simulink model "brainstorm_service"  (R2024a)
settings: Solver=FixedStepDiscrete  StartTime=0.0  StopTime=10.0  RelTol=1e-3
model workspace (MAT data in the model file):
  Anatomy = Simulink.ServiceBus
  Anatomy.Elements_internal(1) = Simulink.FunctionElement
  Anatomy.Elements_internal(1).Prototype = 'GetSubjectMri(bst_fullfile,sessFolders,anat)'
  Anatomy.Elements_internal(1).Name = 'GetSubjectMri'
  Anatomy.Elements_internal(1).Asynchronous = 0
  Anatomy.Elements_internal(1).Arguments(1) = Simulink.BusElement
  Anatomy.Elements_internal(1).Arguments(1).DimensionsMode = 'Fixed'
  Anatomy.Elements_internal(1).Arguments(1).SamplingMode = 'Sample based'
  Anatomy.Elements_internal(1).Arguments(1).SampleTime = -1
  Anatomy.Elements_internal(1).Arguments(1).Name = 'bst_fullfile'
  Anatomy.Elements_internal(1).Arguments(1).DataType_internal = 'double'
  Anatomy.Elements_internal(1).Arguments(1).Complexity = 'real'
  Anatomy.Elements_internal(1).Arguments(1).Dimensions = 1
  Anatomy.Elements_internal(1).Arguments(2) = Simulink.BusElement
  Anatomy.Elements_internal(1).Arguments(2).DimensionsMode = 'Fixed'
  Anatomy.Elements_internal(1).Arguments(2).SamplingMode = 'Sample based'
  Anatomy.Elements_internal(1).Arguments(2).SampleTime = -1
  Anatomy.Elements_internal(1).Arguments(2).Name = 'sessFolders'
  Anatomy.Elements_internal(1).Arguments(2).DataType_internal = 'double'
  Anatomy.Elements_internal(1).Arguments(2).Complexity = 'real'
  Anatomy.Elements_internal(1).Arguments(2).Dimensions = 1
  Anatomy.Elements_internal(1).Arguments(3) = Simulink.BusElement
  Anatomy.Elements_internal(1).Arguments(3).DimensionsMode = 'Fixed'
  Anatomy.Elements_internal(1).Arguments(3).SamplingMode = 'Sample based'
  Anatomy.Elements_internal(1).Arguments(3).SampleTime = -1
  Anatomy.Elements_internal(1).Arguments(3).Name = 'anat'
  Anatomy.Elements_internal(1).Arguments(3).DataType_internal = 'double'
  Anatomy.Elements_internal(1).Arguments(3).Complexity = 'real'
  Anatomy.Elements_internal(1).Arguments(3).Dimensions = 1
  Anatomy.Elements_internal(2) = Simulink.FunctionElement
  Anatomy.Elements_internal(2).Prototype = 'SubjectMriFiles()'
  Anatomy.Elements_internal(2).Name = 'SubjectMriFiles'
  Anatomy.Elements_internal(2).Asynchronous = 0
  coregister = Simulink.ServiceBus
  coregister.Elements_internal = Simulink.FunctionElement
  coregister.Elements_internal.Prototype = 'GetFiducials(json,voxel)'
  coregister.Elements_internal.Name = 'GetFiducials'
  coregister.Elements_internal.Asynchronous = 0
  coregister.Elements_internal.Arguments(1) = Simulink.BusElement
  coregister.Elements_internal.Arguments(1).DimensionsMode = 'Fixed'
  coregister.Elements_internal.Arguments(1).SamplingMode = 'Sample based'
  coregister.Elements_internal.Arguments(1).SampleTime = -1
  coregister.Elements_internal.Arguments(1).Name = 'json'
  coregister.Elements_internal.Arguments(1).DataType_internal = 'double'
  coregister.Elements_internal.Arguments(1).Complexity = 'real'
  coregister.Elements_internal.Arguments(1).Dimensions = 1
  coregister.Elements_internal.Arguments(2) = Simulink.BusElement
  coregister.Elements_internal.Arguments(2).DimensionsMode = 'Fixed'
  coregister.Elements_internal.Arguments(2).SamplingMode = 'Sample based'
  coregister.Elements_internal.Arguments(2).SampleTime = -1
  coregister.Elements_internal.Arguments(2).Name = 'voxel'
  coregister.Elements_internal.Arguments(2).DataType_internal = 'double'
  coregister.Elements_internal.Arguments(2).Complexity = 'real'
  coregister.Elements_internal.Arguments(2).Dimensions = 1
  filePaths = Simulink.ServiceBus
  filePaths.Elements_internal(1) = Simulink.FunctionElement
  filePaths.Elements_internal(1).Prototype = 'bst_fullfile(fPath,fBase,json)'
  filePaths.Elements_internal(1).Name = 'bst_fullfile'
  filePaths.Elements_internal(1).Asynchronous = 0
  filePaths.Elements_internal(1).Arguments(1) = Simulink.BusElement
  filePaths.Elements_internal(1).Arguments(1).DimensionsMode = 'Fixed'
  filePaths.Elements_internal(1).Arguments(1).SamplingMode = 'Sample based'
  filePaths.Elements_internal(1).Arguments(1).SampleTime = -1
  filePaths.Elements_internal(1).Arguments(1).Name = 'fPath'
  filePaths.Elements_internal(1).Arguments(1).DataType_internal = 'double'
  filePaths.Elements_internal(1).Arguments(1).Complexity = 'real'
  filePaths.Elements_internal(1).Arguments(1).Dimensions = 1
  filePaths.Elements_internal(1).Arguments(2) = Simulink.BusElement
  filePaths.Elements_internal(1).Arguments(2).DimensionsMode = 'Fixed'
  filePaths.Elements_internal(1).Arguments(2).SamplingMode = 'Sample based'
  filePaths.Elements_internal(1).Arguments(2).SampleTime = -1
  filePaths.Elements_internal(1).Arguments(2).Name = 'fBase'
  filePaths.Elements_internal(1).Arguments(2).DataType_internal = 'double'
  filePaths.Elements_internal(1).Arguments(2).Complexity = 'real'
  filePaths.Elements_internal(1).Arguments(2).Dimensions = 1
  filePaths.Elements_internal(1).Arguments(3) = Simulink.BusElement
  filePaths.Elements_internal(1).Arguments(3).DimensionsMode = 'Fixed'
  filePaths.Elements_internal(1).Arguments(3).SamplingMode = 'Sample based'
  filePaths.Elements_internal(1).Arguments(3).SampleTime = -1
  filePaths.Elements_internal(1).Arguments(3).Name = 'json'
  filePaths.Elements_internal(1).Arguments(3).DataType_internal = 'double'
  filePaths.Elements_internal(1).Arguments(3).Complexity = 'real'
  filePaths.Elements_internal(1).Arguments(3).Dimensions = 1
  filePaths.Elements_internal(2) = Simulink.FunctionElement
  filePaths.Elements_internal(2).Prototype = 'bst_fileparts()'
  filePaths.Elements_internal(2).Name = 'bst_fileparts'
  filePaths.Elements_internal(2).Asynchronous = 0
  importVolume = Simulink.ServiceBus
  importVolume.Elements_internal(1) = Simulink.FunctionElement
  importVolume.Elements_internal(1).Prototype = 'process_import_bids(ImportBidsDataset)'
  importVolume.Elements_internal(1).Name = 'process_import_bids'
  importVolume.Elements_internal(1).Asynchronous = 0
  importVolume.Elements_internal(1).Arguments = Simulink.BusElement
  importVolume.Elements_internal(1).Arguments.DimensionsMode = 'Fixed'
  importVolume.Elements_internal(1).Arguments.SamplingMode = 'Sample based'
  importVolume.Elements_internal(1).Arguments.SampleTime = -1
  importVolume.Elements_internal(1).Arguments.Name = 'ImportBidsDataset'
  importVolume.Elements_internal(1).Arguments.DataType_internal = 'double'
  importVolume.Elements_internal(1).Arguments.Complexity = 'real'
  importVolume.Elements_internal(1).Arguments.Dimensions = 1
  importVolume.Elements_internal(2) = Simulink.FunctionElement
  importVolume.Elements_internal(2).Prototype = 'ImportBidsDataset(BidsDir,OPTIONS)'
  importVolume.Elements_internal(2).Name = 'ImportBidsDataset'
  importVolume.Elements_internal(2).Asynchronous = 0
  importVolume.Elements_internal(2).Arguments(1) = Simulink.BusElement
  importVolume.Elements_internal(2).Arguments(1).DimensionsMode = 'Fixed'
  importVolume.Elements_internal(2).Arguments(1).SamplingMode = 'Sample based'
  importVolume.Elements_internal(2).Arguments(1).SampleTime = -1
  importVolume.Elements_internal(2).Arguments(1).Name = 'BidsDir'
  importVolume.Elements_internal(2).Arguments(1).DataType_internal = 'double'
  importVolume.Elements_internal(2).Arguments(1).Complexity = 'real'
  importVolume.Elements_internal(2).Arguments(1).Dimensions = 1
  importVolume.Elements_internal(2).Arguments(2) = Simulink.BusElement
  importVolume.Elements_internal(2).Arguments(2).DimensionsMode = 'Fixed'
  importVolume.Elements_internal(2).Arguments(2).SamplingMode = 'Sample based'
  importVolume.Elements_internal(2).Arguments(2).SampleTime = -1
  importVolume.Elements_internal(2).Arguments(2).Name = 'OPTIONS'
  importVolume.Elements_internal(2).Arguments(2).DataType_internal = 'double'
  importVolume.Elements_internal(2).Arguments(2).Complexity = 'real'
  importVolume.Elements_internal(2).Arguments(2).Dimensions = 1
  importVolume.Elements_internal(3) = Simulink.FunctionElement
  importVolume.Elements_internal(3).Prototype = 'GetSubjectMri(bst_fullfile,sessFolders,isess,anat)'
  importVolume.Elements_internal(3).Name = 'GetSubjectMri'
  importVolume.Elements_internal(3).Asynchronous = 0
  importVolume.Elements_internal(3).Arguments(1) = Simulink.BusElement
  importVolume.Elements_internal(3).Arguments(1).DimensionsMode = 'Fixed'
  importVolume.Elements_internal(3).Arguments(1).SamplingMode = 'Sample based'
  importVolume.Elements_internal(3).Arguments(1).SampleTime = -1
  importVolume.Elements_internal(3).Arguments(1).Name = 'bst_fullfile'
  importVolume.Elements_internal(3).Arguments(1).DataType_internal = 'double'
  importVolume.Elements_internal(3).Arguments(1).Complexity = 'real'
  importVolume.Elements_internal(3).Arguments(1).Dimensions = 1
  importVolume.Elements_internal(3).Arguments(2) = Simulink.BusElement
  importVolume.Elements_internal(3).Arguments(2).DimensionsMode = 'Fixed'
  importVolume.Elements_internal(3).Arguments(2).SamplingMode = 'Sample based'
  importVolume.Elements_internal(3).Arguments(2).SampleTime = -1
  importVolume.Elements_internal(3).Arguments(2).Name = 'sessFolders'
  importVolume.Elements_internal(3).Arguments(2).DataType_internal = 'double'
  importVolume.Elements_internal(3).Arguments(2).Complexity = 'real'
  importVolume.Elements_internal(3).Arguments(2).Dimensions = 1
  importVolume.Elements_internal(3).Arguments(3) = Simulink.BusElement
  importVolume.Elements_internal(3).Arguments(3).DimensionsMode = 'Fixed'
  importVolume.Elements_internal(3).Arguments(3).SamplingMode = 'Sample based'
  importVolume.Elements_internal(3).Arguments(3).SampleTime = -1
  importVolume.Elements_internal(3).Arguments(3).Name = 'isess'
  importVolume.Elements_internal(3).Arguments(3).DataType_internal = 'double'
  importVolume.Elements_internal(3).Arguments(3).Complexity = 'real'
  importVolume.Elements_internal(3).Arguments(3).Dimensions = 1
  importVolume.Elements_internal(3).Arguments(4) = Simulink.BusElement
  importVolume.Elements_internal(3).Arguments(4).DimensionsMode = 'Fixed'
  importVolume.Elements_internal(3).Arguments(4).SamplingMode = 'Sample based'
  importVolume.Elements_internal(3).Arguments(4).SampleTime = -1
  importVolume.Elements_internal(3).Arguments(4).Name = 'anat'
  importVolume.Elements_internal(3).Arguments(4).DataType_internal = 'double'
  importVolume.Elements_internal(3).Arguments(4).Complexity = 'real'
  importVolume.Elements_internal(3).Arguments(4).Dimensions = 1
  importVolume.Elements_internal(4) = Simulink.FunctionElement
  importVolume.Elements_internal(4).Prototype = 'GetSubjectSeg(BidsDir,subjName,sessDir,isess,name)'
  importVolume.Elements_internal(4).Name = 'GetSubjectSeg'
  importVolume.Elements_internal(4).Asynchronous = 0
  importVolume.Elements_internal(4).Arguments(1) = Simulink.BusElement
  importVolume.Elements_internal(4).Arguments(1).DimensionsMode = 'Fixed'
  importVolume.Elements_internal(4).Arguments(1).SamplingMode = 'Sample based'
  importVolume.Elements_internal(4).Arguments(1).SampleTime = -1
  importVolume.Elements_internal(4).Arguments(1).Name = 'BidsDir'
  importVolume.Elements_internal(4).Arguments(1).DataType_internal = 'double'
  importVolume.Elements_internal(4).Arguments(1).Complexity = 'real'
  importVolume.Elements_internal(4).Arguments(1).Dimensions = 1
  importVolume.Elements_internal(4).Arguments(2) = Simulink.BusElement
  importVolume.Elements_internal(4).Arguments(2).DimensionsMode = 'Fixed'
  importVolume.Elements_internal(4).Arguments(2).SamplingMode = 'Sample based'
  importVolume.Elements_internal(4).Arguments(2).SampleTime = -1
  importVolume.Elements_internal(4).Arguments(2).Name = 'subjName'
  importVolume.Elements_internal(4).Arguments(2).DataType_internal = 'double'
  importVolume.Elements_internal(4).Arguments(2).Complexity = 'real'
  importVolume.Elements_internal(4).Arguments(2).Dimensions = 1
  importVolume.Elements_internal(4).Arguments(3) = Simulink.BusElement
  importVolume.Elements_internal(4).Arguments(3).DimensionsMode = 'Fixed'
  importVolume.Elements_internal(4).Arguments(3).SamplingMode = 'Sample based'
  importVolume.Elements_internal(4).Arguments(3).SampleTime = -1
  importVolume.Elements_internal(4).Arguments(3).Name = 'sessDir'
  importVolume.Elements_internal(4).Arguments(3).DataType_internal = 'double'
  importVolume.Elements_internal(4).Arguments(3).Complexity = 'real'
  importVolume.Elements_internal(4).Arguments(3).Dimensions = 1
  importVolume.Elements_internal(4).Arguments(4) = Simulink.BusElement
  importVolume.Elements_internal(4).Arguments(4).DimensionsMode = 'Fixed'
  importVolume.Elements_internal(4).Arguments(4).SamplingMode = 'Sample based'
  importVolume.Elements_internal(4).Arguments(4).SampleTime = -1
  importVolume.Elements_internal(4).Arguments(4).Name = 'isess'
  importVolume.Elements_internal(4).Arguments(4).DataType_internal = 'double'
  importVolume.Elements_internal(4).Arguments(4).Complexity = 'real'
  importVolume.Elements_internal(4).Arguments(4).Dimensions = 1
  importVolume.Elements_internal(4).Arguments(5) = Simulink.BusElement
  importVolume.Elements_internal(4).Arguments(5).DimensionsMode = 'Fixed'
  importVolume.Elements_internal(4).Arguments(5).SamplingMode = 'Sample based'
  importVolume.Elements_internal(4).Arguments(5).SampleTime = -1
  importVolume.Elements_internal(4).Arguments(5).Name = 'name'
  importVolume.Elements_internal(4).Arguments(5).DataType_internal = 'double'
  importVolume.Elements_internal(4).Arguments(5).Complexity = 'real'
  importVolume.Elements_internal(4).Arguments(5).Dimensions = 1
settings Model: Creator=diell  LastModifiedBy=diell

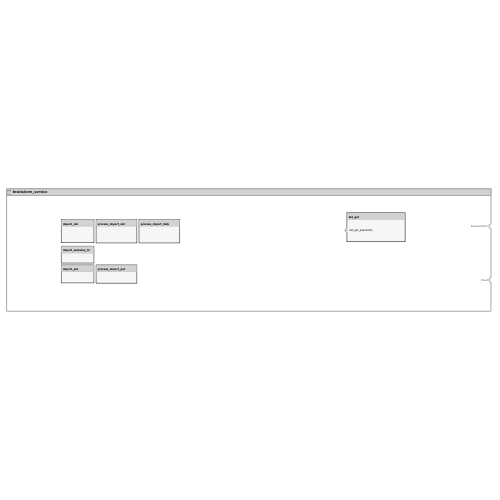
[thumbnail: Simulink's stored preview of the top-level diagram]
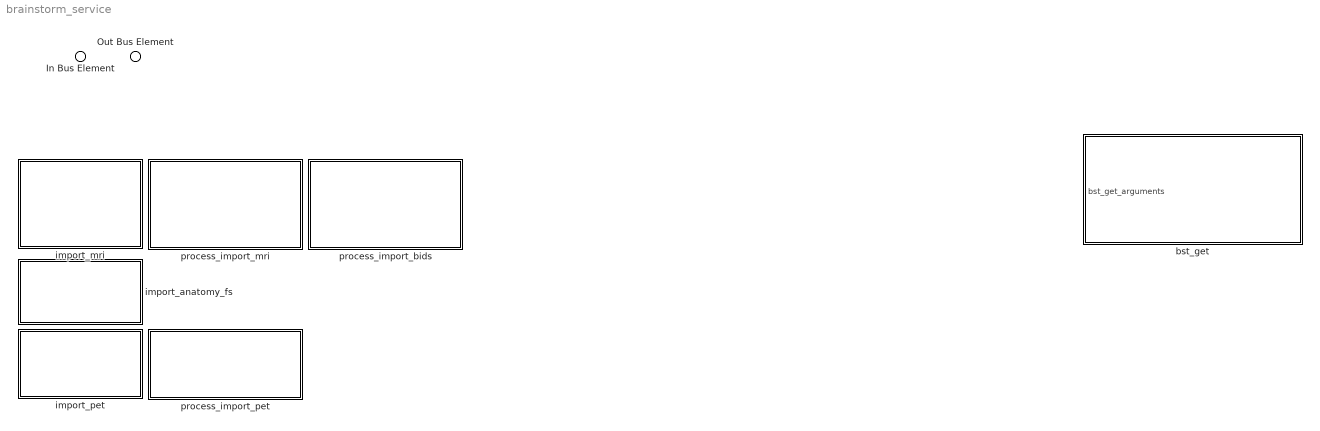
== system brainstorm_service ==
  In Bus Element : Inport  AllowServiceAccess=on  PortName=Client
  bst_get : Subsystem
      settings: PortSchema="{\"entries\":[{\"content\":{\"headerSize\":26,\"margin\":15,\"minimumSpacing\":25,\"sides\":[{\"content\":{\"connectorIds\":[\"In1\"]},\"type\":\"ConnectorPlacement.EquallySpacedRectSide\",\"uuid\":\"7074e736-93ca-48e6-9107-0c0acde2c1e1\"},{\"content\":{\"side\":\"RIGHT\"},\"type\":\"ConnectorPlacement.EquallySpacedRectSide\",\"uuid\":\"49ca3538-4b0a-47e3-9b9f-d0d67086357c\"},{\"content\":{\"side\":\"TOP\"},\"type\":\"ConnectorPlacement.EquallySpacedRectSide\",\"uuid\":\"104f6ef2-0cbf-4c6c-8b7e-db8a41d08c3b\"}]},\"type\":\"ConnectorPlacement.EquallySpacedConnector\",\"uuid\":\"4cd04038-0b55-4958-ad0a-aa155b20eca4\"}],\"packageUris\":[\"http://schema.mathworks.com/mf0/Connector/R2020b\"],\"version\":\"1.0\"}"
  import_anatomy_fs : Subsystem
      settings: PortSchema="{\"entries\":[{\"content\":{\"headerSize\":26,\"margin\":15,\"minimumSpacing\":25,\"sides\":[{\"content\":{},\"type\":\"ConnectorPlacement.EquallySpacedRectSide\",\"uuid\":\"7be748b9-e2b2-4fca-9238-079eea30a187\"},{\"content\":{\"side\":\"RIGHT\"},\"type\":\"ConnectorPlacement.EquallySpacedRectSide\",\"uuid\":\"1b861973-f2f5-4eed-832d-e933959a74ac\"},{\"content\":{\"side\":\"TOP\"},\"type\":\"ConnectorPlacement.EquallySpacedRectSide\",\"uuid\":\"dbbefc62-cbb0-405a-aca0-d0e93444e038\"}]},\"type\":\"ConnectorPlacement.EquallySpacedConnector\",\"uuid\":\"452c4985-6d59-43c7-a9cf-3ab3814160fd\"}],\"packageUris\":[\"http://schema.mathworks.com/mf0/Connector/R2020b\"],\"version\":\"1.0\"}"
  import_mri : Subsystem
      settings: PortSchema="{\"entries\":[{\"content\":{\"headerSize\":26,\"margin\":15,\"minimumSpacing\":25,\"sides\":[{\"content\":{},\"type\":\"ConnectorPlacement.EquallySpacedRectSide\",\"uuid\":\"7be748b9-e2b2-4fca-9238-079eea30a187\"},{\"content\":{\"side\":\"RIGHT\"},\"type\":\"ConnectorPlacement.EquallySpacedRectSide\",\"uuid\":\"1b861973-f2f5-4eed-832d-e933959a74ac\"},{\"content\":{\"side\":\"TOP\"},\"type\":\"ConnectorPlacement.EquallySpacedRectSide\",\"uuid\":\"dbbefc62-cbb0-405a-aca0-d0e93444e038\"}]},\"type\":\"ConnectorPlacement.EquallySpacedConnector\",\"uuid\":\"452c4985-6d59-43c7-a9cf-3ab3814160fd\"}],\"packageUris\":[\"http://schema.mathworks.com/mf0/Connector/R2020b\"],\"version\":\"1.0\"}"
  import_pet : Subsystem
      settings: PortSchema="{\"entries\":[{\"content\":{\"headerSize\":26,\"margin\":15,\"minimumSpacing\":25,\"sides\":[{\"content\":{},\"type\":\"ConnectorPlacement.EquallySpacedRectSide\",\"uuid\":\"7be748b9-e2b2-4fca-9238-079eea30a187\"},{\"content\":{\"side\":\"RIGHT\"},\"type\":\"ConnectorPlacement.EquallySpacedRectSide\",\"uuid\":\"1b861973-f2f5-4eed-832d-e933959a74ac\"},{\"content\":{\"side\":\"TOP\"},\"type\":\"ConnectorPlacement.EquallySpacedRectSide\",\"uuid\":\"dbbefc62-cbb0-405a-aca0-d0e93444e038\"}]},\"type\":\"ConnectorPlacement.EquallySpacedConnector\",\"uuid\":\"452c4985-6d59-43c7-a9cf-3ab3814160fd\"}],\"packageUris\":[\"http://schema.mathworks.com/mf0/Connector/R2020b\"],\"version\":\"1.0\"}"
  process_import_bids : Subsystem
      settings: PortSchema="{\"entries\":[{\"content\":{\"headerSize\":26,\"margin\":15,\"minimumSpacing\":25,\"sides\":[{\"content\":{},\"type\":\"ConnectorPlacement.EquallySpacedRectSide\",\"uuid\":\"7be748b9-e2b2-4fca-9238-079eea30a187\"},{\"content\":{\"side\":\"RIGHT\"},\"type\":\"ConnectorPlacement.EquallySpacedRectSide\",\"uuid\":\"1b861973-f2f5-4eed-832d-e933959a74ac\"},{\"content\":{\"side\":\"TOP\"},\"type\":\"ConnectorPlacement.EquallySpacedRectSide\",\"uuid\":\"dbbefc62-cbb0-405a-aca0-d0e93444e038\"}]},\"type\":\"ConnectorPlacement.EquallySpacedConnector\",\"uuid\":\"452c4985-6d59-43c7-a9cf-3ab3814160fd\"}],\"packageUris\":[\"http://schema.mathworks.com/mf0/Connector/R2020b\"],\"version\":\"1.0\"}"
  process_import_mri : Subsystem
      settings: PortSchema="{\"entries\":[{\"content\":{\"headerSize\":26,\"margin\":15,\"minimumSpacing\":25,\"sides\":[{\"content\":{},\"type\":\"ConnectorPlacement.EquallySpacedRectSide\",\"uuid\":\"7be748b9-e2b2-4fca-9238-079eea30a187\"},{\"content\":{\"side\":\"RIGHT\"},\"type\":\"ConnectorPlacement.EquallySpacedRectSide\",\"uuid\":\"1b861973-f2f5-4eed-832d-e933959a74ac\"},{\"content\":{\"side\":\"TOP\"},\"type\":\"ConnectorPlacement.EquallySpacedRectSide\",\"uuid\":\"dbbefc62-cbb0-405a-aca0-d0e93444e038\"}]},\"type\":\"ConnectorPlacement.EquallySpacedConnector\",\"uuid\":\"452c4985-6d59-43c7-a9cf-3ab3814160fd\"}],\"packageUris\":[\"http://schema.mathworks.com/mf0/Connector/R2020b\"],\"version\":\"1.0\"}"
  process_import_pet : Subsystem
      settings: PortSchema="{\"entries\":[{\"content\":{\"headerSize\":26,\"margin\":15,\"minimumSpacing\":25,\"sides\":[{\"content\":{},\"type\":\"ConnectorPlacement.EquallySpacedRectSide\",\"uuid\":\"7be748b9-e2b2-4fca-9238-079eea30a187\"},{\"content\":{\"side\":\"RIGHT\"},\"type\":\"ConnectorPlacement.EquallySpacedRectSide\",\"uuid\":\"1b861973-f2f5-4eed-832d-e933959a74ac\"},{\"content\":{\"side\":\"TOP\"},\"type\":\"ConnectorPlacement.EquallySpacedRectSide\",\"uuid\":\"dbbefc62-cbb0-405a-aca0-d0e93444e038\"}]},\"type\":\"ConnectorPlacement.EquallySpacedConnector\",\"uuid\":\"452c4985-6d59-43c7-a9cf-3ab3814160fd\"}],\"packageUris\":[\"http://schema.mathworks.com/mf0/Connector/R2020b\"],\"version\":\"1.0\"}"
  Out Bus Element : Outport  PortName=brainstormEnv

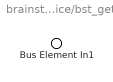
== system brainstorm_service/bst_get ==
  Bus Element In1 : Inport  PortName=bst_get_arguments

== system brainstorm_service/import_anatomy_fs ==

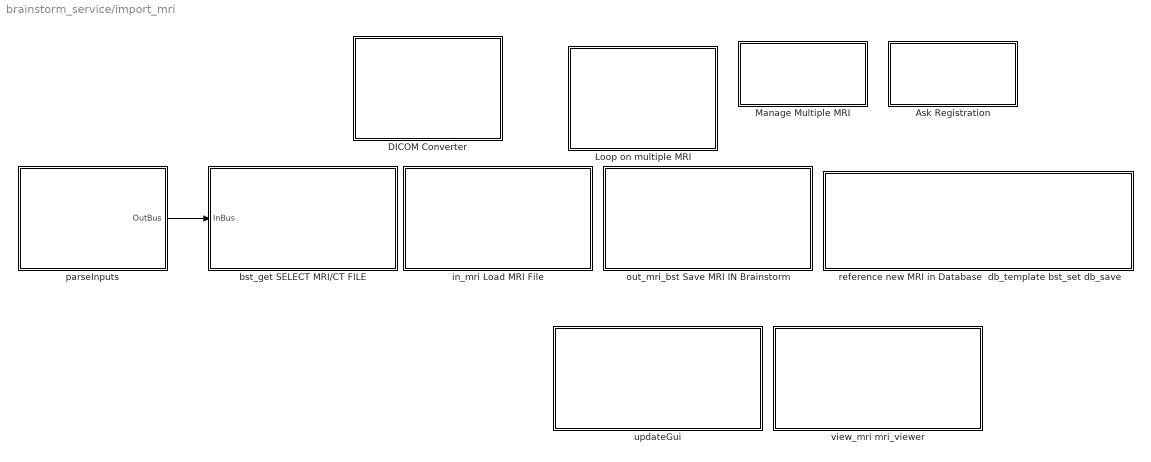
== system brainstorm_service/import_mri ==
  Ask Registration : Subsystem
      settings: PortSchema="{\"entries\":[{\"content\":{\"headerSize\":26,\"margin\":15,\"minimumSpacing\":25,\"sides\":[{\"content\":{},\"type\":\"ConnectorPlacement.EquallySpacedRectSide\",\"uuid\":\"7be748b9-e2b2-4fca-9238-079eea30a187\"},{\"content\":{\"side\":\"RIGHT\"},\"type\":\"ConnectorPlacement.EquallySpacedRectSide\",\"uuid\":\"1b861973-f2f5-4eed-832d-e933959a74ac\"},{\"content\":{\"side\":\"TOP\"},\"type\":\"ConnectorPlacement.EquallySpacedRectSide\",\"uuid\":\"dbbefc62-cbb0-405a-aca0-d0e93444e038\"}]},\"type\":\"ConnectorPlacement.EquallySpacedConnector\",\"uuid\":\"452c4985-6d59-43c7-a9cf-3ab3814160fd\"}],\"packageUris\":[\"http://schema.mathworks.com/mf0/Connector/R2020b\"],\"version\":\"1.0\"}"
  DICOM Converter : Subsystem
      settings: PortSchema="{\"entries\":[{\"content\":{\"headerSize\":26,\"margin\":15,\"minimumSpacing\":25,\"sides\":[{\"content\":{},\"type\":\"ConnectorPlacement.EquallySpacedRectSide\",\"uuid\":\"7be748b9-e2b2-4fca-9238-079eea30a187\"},{\"content\":{\"side\":\"RIGHT\"},\"type\":\"ConnectorPlacement.EquallySpacedRectSide\",\"uuid\":\"1b861973-f2f5-4eed-832d-e933959a74ac\"},{\"content\":{\"side\":\"TOP\"},\"type\":\"ConnectorPlacement.EquallySpacedRectSide\",\"uuid\":\"dbbefc62-cbb0-405a-aca0-d0e93444e038\"}]},\"type\":\"ConnectorPlacement.EquallySpacedConnector\",\"uuid\":\"452c4985-6d59-43c7-a9cf-3ab3814160fd\"}],\"packageUris\":[\"http://schema.mathworks.com/mf0/Connector/R2020b\"],\"version\":\"1.0\"}"
  Loop on multiple MRI : Subsystem
      settings: PortSchema="{\"entries\":[{\"content\":{\"headerSize\":26,\"margin\":15,\"minimumSpacing\":25,\"sides\":[{\"content\":{},\"type\":\"ConnectorPlacement.EquallySpacedRectSide\",\"uuid\":\"7be748b9-e2b2-4fca-9238-079eea30a187\"},{\"content\":{\"side\":\"RIGHT\"},\"type\":\"ConnectorPlacement.EquallySpacedRectSide\",\"uuid\":\"1b861973-f2f5-4eed-832d-e933959a74ac\"},{\"content\":{\"side\":\"TOP\"},\"type\":\"ConnectorPlacement.EquallySpacedRectSide\",\"uuid\":\"dbbefc62-cbb0-405a-aca0-d0e93444e038\"}]},\"type\":\"ConnectorPlacement.EquallySpacedConnector\",\"uuid\":\"452c4985-6d59-43c7-a9cf-3ab3814160fd\"}],\"packageUris\":[\"http://schema.mathworks.com/mf0/Connector/R2020b\"],\"version\":\"1.0\"}"
  Manage Multiple MRI : Subsystem
      settings: PortSchema="{\"entries\":[{\"content\":{\"headerSize\":26,\"margin\":15,\"minimumSpacing\":25,\"sides\":[{\"content\":{},\"type\":\"ConnectorPlacement.EquallySpacedRectSide\",\"uuid\":\"7be748b9-e2b2-4fca-9238-079eea30a187\"},{\"content\":{\"side\":\"RIGHT\"},\"type\":\"ConnectorPlacement.EquallySpacedRectSide\",\"uuid\":\"1b861973-f2f5-4eed-832d-e933959a74ac\"},{\"content\":{\"side\":\"TOP\"},\"type\":\"ConnectorPlacement.EquallySpacedRectSide\",\"uuid\":\"dbbefc62-cbb0-405a-aca0-d0e93444e038\"}]},\"type\":\"ConnectorPlacement.EquallySpacedConnector\",\"uuid\":\"452c4985-6d59-43c7-a9cf-3ab3814160fd\"}],\"packageUris\":[\"http://schema.mathworks.com/mf0/Connector/R2020b\"],\"version\":\"1.0\"}"
  bst_get SELECT MRI/CT FILE : Subsystem
      settings: PortSchema="{\"entries\":[{\"content\":{\"headerSize\":26,\"margin\":15,\"minimumSpacing\":25,\"sides\":[{\"content\":{\"connectorIds\":[\"In1\"]},\"type\":\"ConnectorPlacement.EquallySpacedRectSide\",\"uuid\":\"7be748b9-e2b2-4fca-9238-079eea30a187\"},{\"content\":{\"side\":\"RIGHT\"},\"type\":\"ConnectorPlacement.EquallySpacedRectSide\",\"uuid\":\"1b861973-f2f5-4eed-832d-e933959a74ac\"},{\"content\":{\"side\":\"TOP\"},\"type\":\"ConnectorPlacement.EquallySpacedRectSide\",\"uuid\":\"dbbefc62-cbb0-405a-aca0-d0e93444e038\"}]},\"type\":\"ConnectorPlacement.EquallySpacedConnector\",\"uuid\":\"452c4985-6d59-43c7-a9cf-3ab3814160fd\"}],\"packageUris\":[\"http://schema.mathworks.com/mf0/Connector/R2020b\"],\"version\":\"1.0\"}"
  in_mri Load MRI File : Subsystem
      settings: PortSchema="{\"entries\":[{\"content\":{\"headerSize\":26,\"margin\":15,\"minimumSpacing\":25,\"sides\":[{\"content\":{},\"type\":\"ConnectorPlacement.EquallySpacedRectSide\",\"uuid\":\"7be748b9-e2b2-4fca-9238-079eea30a187\"},{\"content\":{\"side\":\"RIGHT\"},\"type\":\"ConnectorPlacement.EquallySpacedRectSide\",\"uuid\":\"1b861973-f2f5-4eed-832d-e933959a74ac\"},{\"content\":{\"side\":\"TOP\"},\"type\":\"ConnectorPlacement.EquallySpacedRectSide\",\"uuid\":\"dbbefc62-cbb0-405a-aca0-d0e93444e038\"}]},\"type\":\"ConnectorPlacement.EquallySpacedConnector\",\"uuid\":\"452c4985-6d59-43c7-a9cf-3ab3814160fd\"}],\"packageUris\":[\"http://schema.mathworks.com/mf0/Connector/R2020b\"],\"version\":\"1.0\"}"
  out_mri_bst Save MRI IN Brainstorm : Subsystem
      settings: PortSchema="{\"entries\":[{\"content\":{\"headerSize\":26,\"margin\":15,\"minimumSpacing\":25,\"sides\":[{\"content\":{},\"type\":\"ConnectorPlacement.EquallySpacedRectSide\",\"uuid\":\"7be748b9-e2b2-4fca-9238-079eea30a187\"},{\"content\":{\"side\":\"RIGHT\"},\"type\":\"ConnectorPlacement.EquallySpacedRectSide\",\"uuid\":\"1b861973-f2f5-4eed-832d-e933959a74ac\"},{\"content\":{\"side\":\"TOP\"},\"type\":\"ConnectorPlacement.EquallySpacedRectSide\",\"uuid\":\"dbbefc62-cbb0-405a-aca0-d0e93444e038\"}]},\"type\":\"ConnectorPlacement.EquallySpacedConnector\",\"uuid\":\"452c4985-6d59-43c7-a9cf-3ab3814160fd\"}],\"packageUris\":[\"http://schema.mathworks.com/mf0/Connector/R2020b\"],\"version\":\"1.0\"}"
  parseInputs : Subsystem
      settings: PortSchema="{\"entries\":[{\"content\":{\"headerSize\":26,\"margin\":15,\"minimumSpacing\":25,\"sides\":[{\"content\":{},\"type\":\"ConnectorPlacement.EquallySpacedRectSide\",\"uuid\":\"7be748b9-e2b2-4fca-9238-079eea30a187\"},{\"content\":{\"connectorIds\":[\"Out1\"],\"side\":\"RIGHT\"},\"type\":\"ConnectorPlacement.EquallySpacedRectSide\",\"uuid\":\"1b861973-f2f5-4eed-832d-e933959a74ac\"},{\"content\":{\"side\":\"TOP\"},\"type\":\"ConnectorPlacement.EquallySpacedRectSide\",\"uuid\":\"dbbefc62-cbb0-405a-aca0-d0e93444e038\"}]},\"type\":\"ConnectorPlacement.EquallySpacedConnector\",\"uuid\":\"452c4985-6d59-43c7-a9cf-3ab3814160fd\"}],\"packageUris\":[\"http://schema.mathworks.com/mf0/Connector/R2020b\"],\"version\":\"1.0\"}"
  reference new MRI in Database  db_template bst_set db_save : Subsystem
      settings: PortSchema="{\"entries\":[{\"content\":{\"headerSize\":26,\"margin\":15,\"minimumSpacing\":25,\"sides\":[{\"content\":{},\"type\":\"ConnectorPlacement.EquallySpacedRectSide\",\"uuid\":\"7be748b9-e2b2-4fca-9238-079eea30a187\"},{\"content\":{\"side\":\"RIGHT\"},\"type\":\"ConnectorPlacement.EquallySpacedRectSide\",\"uuid\":\"1b861973-f2f5-4eed-832d-e933959a74ac\"},{\"content\":{\"side\":\"TOP\"},\"type\":\"ConnectorPlacement.EquallySpacedRectSide\",\"uuid\":\"dbbefc62-cbb0-405a-aca0-d0e93444e038\"},{\"content\":{\"side\":\"BOTTOM\"},\"type\":\"ConnectorPlacement.EquallySpacedRectSide\",\"uuid\":\"a01a4bc1-e9b9-447b-a64e-1a76c5c75434\"}]},\"type\":\"ConnectorPlacement.EquallySpacedConnector\",\"uuid\":\"452c4985-6d59-43c7-a9cf-3ab3814160fd\"}],\"packageUris\":[\"http://schema.mathworks.com/mf0/Connector/R2020b\"],\"version\":\"1.0\"}"
  updateGui : Subsystem
      settings: PortSchema="{\"entries\":[{\"content\":{\"headerSize\":26,\"margin\":15,\"minimumSpacing\":25,\"sides\":[{\"content\":{},\"type\":\"ConnectorPlacement.EquallySpacedRectSide\",\"uuid\":\"7be748b9-e2b2-4fca-9238-079eea30a187\"},{\"content\":{\"side\":\"RIGHT\"},\"type\":\"ConnectorPlacement.EquallySpacedRectSide\",\"uuid\":\"1b861973-f2f5-4eed-832d-e933959a74ac\"},{\"content\":{\"side\":\"TOP\"},\"type\":\"ConnectorPlacement.EquallySpacedRectSide\",\"uuid\":\"dbbefc62-cbb0-405a-aca0-d0e93444e038\"}]},\"type\":\"ConnectorPlacement.EquallySpacedConnector\",\"uuid\":\"452c4985-6d59-43c7-a9cf-3ab3814160fd\"}],\"packageUris\":[\"http://schema.mathworks.com/mf0/Connector/R2020b\"],\"version\":\"1.0\"}"
  view_mri mri_viewer : Subsystem
      settings: PortSchema="{\"entries\":[{\"content\":{\"headerSize\":26,\"margin\":15,\"minimumSpacing\":25,\"sides\":[{\"content\":{},\"type\":\"ConnectorPlacement.EquallySpacedRectSide\",\"uuid\":\"7be748b9-e2b2-4fca-9238-079eea30a187\"},{\"content\":{\"side\":\"RIGHT\"},\"type\":\"ConnectorPlacement.EquallySpacedRectSide\",\"uuid\":\"1b861973-f2f5-4eed-832d-e933959a74ac\"},{\"content\":{\"side\":\"TOP\"},\"type\":\"ConnectorPlacement.EquallySpacedRectSide\",\"uuid\":\"dbbefc62-cbb0-405a-aca0-d0e93444e038\"}]},\"type\":\"ConnectorPlacement.EquallySpacedConnector\",\"uuid\":\"452c4985-6d59-43c7-a9cf-3ab3814160fd\"}],\"packageUris\":[\"http://schema.mathworks.com/mf0/Connector/R2020b\"],\"version\":\"1.0\"}"
  wires:
  parseInputs/1(OutBus) -> bst_get SELECT MRI/CT FILE/1(InBus)

== system brainstorm_service/import_pet ==

== system brainstorm_service/process_import_bids ==

== system brainstorm_service/process_import_mri ==

== system brainstorm_service/process_import_pet ==

== system brainstorm_service/import_mri/Ask Registration ==

== system brainstorm_service/import_mri/DICOM Converter ==

== system brainstorm_service/import_mri/Loop on multiple MRI ==

== system brainstorm_service/import_mri/Manage Multiple MRI ==

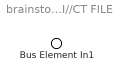
== system brainstorm_service/import_mri/bst_get SELECT MRI//CT FILE ==
  Bus Element In1 : Inport  PortName=InBus

== system brainstorm_service/import_mri/in_mri Load MRI File ==

== system brainstorm_service/import_mri/out_mri_bst Save MRI IN Brainstorm ==

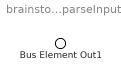
== system brainstorm_service/import_mri/parseInputs ==
  Bus Element Out1 : Outport  PortName=OutBus

== system brainstorm_service/import_mri/reference new MRI in Database  db_template bst_set db_save ==

== system brainstorm_service/import_mri/updateGui ==

== system brainstorm_service/import_mri/view_mri mri_viewer ==
